simulink model "Pole_zero_canc_reg"  (R2023b)
settings: Solver=VariableStepAuto  StartTime=0.0  StopTime=20.0  RelTol=1e-3
values from neighbouring files (symbols this model uses):
  den_phi = cell2mat(G_t2p.Denominator)    [consistent.m]    (also in dyn_model_mark.m)
  den_theta = cell2mat(G_ol.Denominator(1,1))    [consistent.m]    (also in dyn_model_mark.m)
  num_phi = cell2mat(G_t2p.Numerator)    [consistent.m]    (also in dyn_model_mark.m)
  num_theta = cell2mat(G_ol.Numerator(1,1))    [consistent.m]    (also in dyn_model_mark.m)
  Va_bar = double(sol)    [consistent.m]    (also in dyn_model_mark.m)
  x1_bar = 0    [consistent.m]    (also in dyn_model_mark.m)
  x3_bar = 0    [consistent.m]    (also in dyn_model_mark.m = 3.14159265359)
undefined symbols (not defined in the file or in its folder): den_R_phi, den_R_theta, num_R_phi, num_R_theta
libraries: simulink_extras x4
settings Model: Creator=Mark  LastModifiedBy=Mark

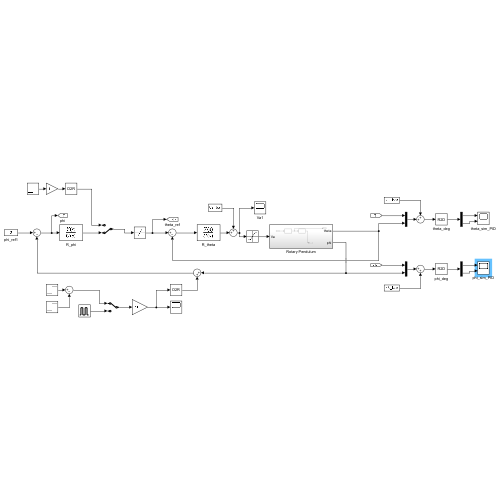
[thumbnail: Simulink's stored preview of the top-level diagram]
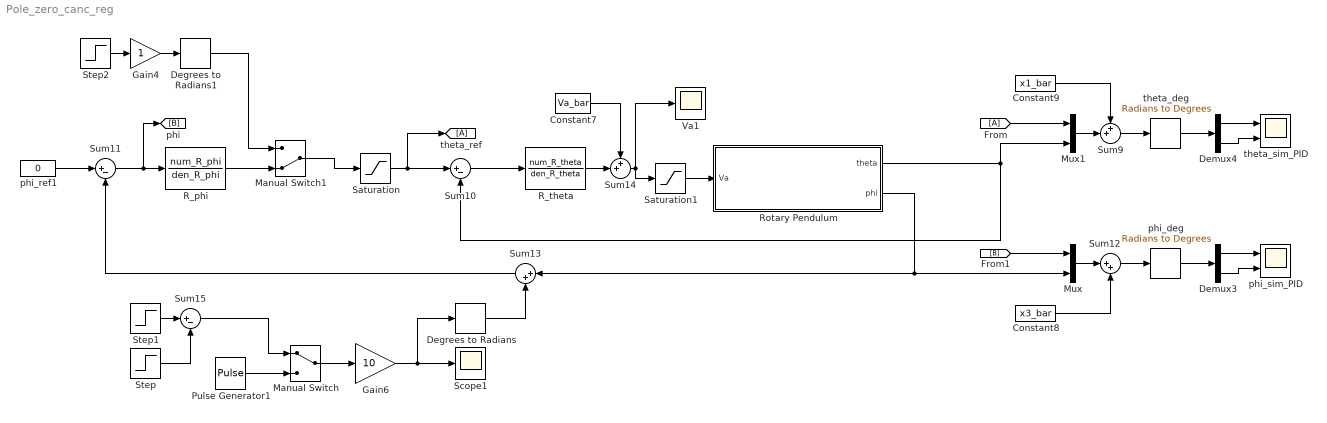
== system Pole_zero_canc_reg ==
  Constant7 : Constant  Value=Va_bar
  Constant8 : Constant  Value=x3_bar
  Constant9 : Constant  Value=x1_bar
  Degrees to Radians : simulink_extras/Transformations/Degrees to Radians
  Degrees to Radians1 : simulink_extras/Transformations/Degrees to Radians
  Demux3 : Demux  Outputs=2
  Demux4 : Demux  Outputs=2
  From : From
  Gain4 : Gain
  Gain6 : Gain  Gain=10
  Manual Switch : ManualSwitch
  Manual Switch1 : ManualSwitch  CurrentSetting=0
  Mux : Mux  Inputs=2
  Mux1 : Mux  Inputs=2
  Pulse Generator1 : DiscretePulseGenerator  PulseType=Time based  Period=10000  PulseWidth=0.005  PhaseDelay=30
  R_phi : TransferFcn  Numerator=num_R_phi  Denominator=den_R_phi
  R_theta : TransferFcn  Numerator=num_R_theta  Denominator=den_R_theta
  Rotary Pendulum : Subsystem
  Saturation : Saturate  UpperLimit=pi/2  LowerLimit=-pi/2
  Saturation1 : Saturate  UpperLimit=10  LowerLimit=-10
  Scope1 : Scope
  Step : Step  Time=1.05  SampleTime=0
  Step1 : Step  SampleTime=0
  Step2 : Step  SampleTime=0
  Sum10 : Sum  Inputs=|+-
  Sum11 : Sum  Inputs=|+-
  Sum12 : Sum  Inputs=|++
  Sum13 : Sum  Inputs=|++
  Sum14 : Sum  Inputs=++|
  Sum15 : Sum  Inputs=|+-
  Sum9 : Sum  Inputs=++|
  Va1 : Scope
  phi_deg : simulink_extras/Transformations/Radians to Degrees
  phi_ref1 : Constant  Value=0
  phi_sim_PID : Scope  NumInputPorts=2
  theta_deg : simulink_extras/Transformations/Radians to Degrees
  theta_ref : Goto
  theta_sim_PID : Scope  NumInputPorts=2
  wires:
  Rotary Pendulum/1(theta) -> Mux1/2, Sum10/2
  Constant8/1 -> Sum12/2
  Saturation/1 -> theta_ref/1, Sum10/1
  Step1/1 -> Sum15/1
  Degrees to Radians1/1 -> Manual Switch1/1
  Rotary Pendulum/2(phi) -> Sum13/1, Mux/2
  Demux3/1 -> phi_sim_PID/1
  Sum15/1 -> Manual Switch/1
  Demux4/2 -> theta_sim_PID/2
  theta_deg/1 -> Demux4/1
  Degrees to Radians/1 -> Sum13/2
  Step/1 -> Sum15/2
  Manual Switch1/1 -> Saturation/1
  Saturation1/1 -> Rotary Pendulum/1(Va)
  Pulse Generator1/1 -> Manual Switch/2
  Demux3/2 -> phi_sim_PID/2
  Mux/1 -> Sum12/1
  Sum14/1 -> Saturation1/1, Va1/1
  phi_deg/1 -> Demux3/1
  Demux4/1 -> theta_sim_PID/1
  Constant7/1 -> Sum14/1
  Constant9/1 -> Sum9/1
  Mux1/1 -> Sum9/2
  R_phi/1 -> Manual Switch1/2
  Manual Switch/1 -> Gain6/1
  From/1 -> Mux1/1
  Sum12/1 -> phi_deg/1
  Gain4/1 -> Degrees to Radians1/1
  Gain6/1 -> Scope1/1, Degrees to Radians/1
  Sum13/1 -> Sum11/2
  R_theta/1 -> Sum14/2
  Sum11/1 -> [B], R_phi/1
  phi_ref1/1 -> Sum11/1
  Sum9/1 -> theta_deg/1
  Step2/1 -> Gain4/1
  Sum10/1 -> R_theta/1
  [B] -> Mux/1

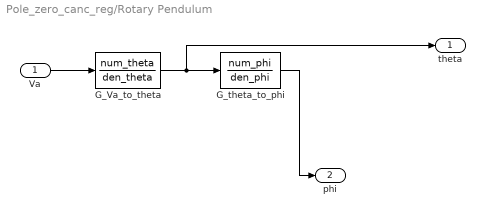
== system Pole_zero_canc_reg/Rotary Pendulum ==
  Va : Inport
  G_Va_to_theta : TransferFcn  Numerator=num_theta  Denominator=den_theta
  G_theta_to_phi : TransferFcn  Numerator=num_phi  Denominator=den_phi
  theta : Outport
  phi : Outport  Port=2
  wires:
  G_theta_to_phi/1 -> phi/1
  G_Va_to_theta/1 -> theta/1, G_theta_to_phi/1
  Va/1 -> G_Va_to_theta/1
